simulink model "control_f86_LQR"  (R2019b)
settings: Solver=VariableStepAuto  StartTime=0.0  StopTime=simtime  RelTol=1e-3
values from neighbouring files (symbols this model uses):
  matrices = matrices_generator(linearization,simtime,T,WIND)    [main.m]    (also in matrices.mat = )
  path =     [path.mat]
  T = 0.021    [main.m]
settings Model: Creator=Usuario  LastModifiedBy=Usuario
settings SolverCC: ZeroCrossAlgorithm=Adaptive  AlgebraicLoopSolver=LineSearch
settings DebuggingCC: MaxConsecutiveZCsMsg=none  IgnoredZcDiagnostic=none  UnderSpecifiedDimensionMsg=warning

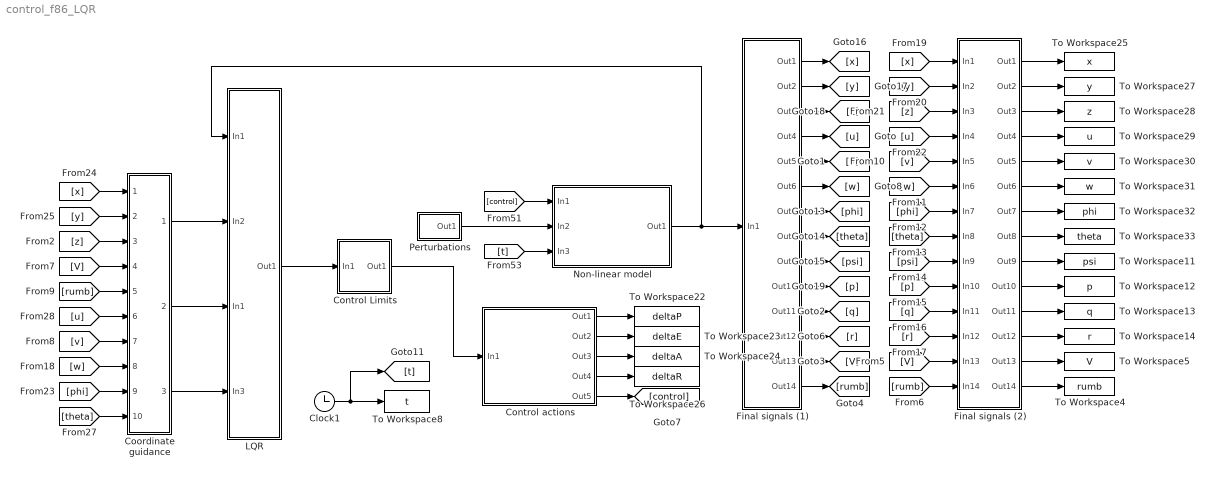
== system control_f86_LQR ==
  Clock1 : Clock
  Control Limits : Subsystem
  Control actions : Subsystem
  Coordinate guidance : Subsystem
  Final signals (1) : Subsystem
  Final signals (2) : Subsystem
  LQR : Subsystem
  Non-linear model : Subsystem
  "Perturbations " : Subsystem
  To Workspace11 : ToWorkspace  VariableName=psi  SampleTime=T
  To Workspace12 : ToWorkspace  VariableName=p  SampleTime=T
  To Workspace13 : ToWorkspace  VariableName=q  SampleTime=T
  To Workspace14 : ToWorkspace  VariableName=r  SampleTime=T
  To Workspace22 : ToWorkspace  VariableName=deltaP  SampleTime=T
  To Workspace23 : ToWorkspace  VariableName=deltaE  SampleTime=T
  To Workspace24 : ToWorkspace  VariableName=deltaA  SampleTime=T
  To Workspace25 : ToWorkspace  VariableName=x  SampleTime=T
  To Workspace26 : ToWorkspace  VariableName=deltaR  SampleTime=T
  To Workspace27 : ToWorkspace  VariableName=y  SampleTime=T
  To Workspace28 : ToWorkspace  VariableName=z  SampleTime=T
  To Workspace29 : ToWorkspace  VariableName=u  SampleTime=T
  To Workspace30 : ToWorkspace  VariableName=v  SampleTime=T
  To Workspace31 : ToWorkspace  VariableName=w  SampleTime=T
  To Workspace32 : ToWorkspace  VariableName=phi  SampleTime=T
  To Workspace33 : ToWorkspace  VariableName=theta  SampleTime=T
  To Workspace4 : ToWorkspace  VariableName=rumb  SampleTime=T
  To Workspace5 : ToWorkspace  VariableName=V  SampleTime=T
  To Workspace8 : ToWorkspace  VariableName=t  SampleTime=T
  wires:
  Non-linear model/1(Out1) -> LQR/1("In1 "), Final signals (1)/1(In1)
  "Perturbations "/1(Out1) -> Non-linear model/2(In2)
  Clock1/1 -> [t], To Workspace8/1
  [control] -> Non-linear model/1(In1)
  [t] -> Non-linear model/3(In3)
  LQR/1(Out1) -> Control Limits/1(In1)
  Control Limits/1(Out1) -> Control actions/1(In1)
  [x] -> Coordinate guidance/1(In1)
  [y] -> Coordinate guidance/2(In2)
  Coordinate guidance/1(Out1) -> LQR/2(In2)
  Coordinate guidance/2(Out2) -> LQR/3(In1)
  Coordinate guidance/3(Out3) -> LQR/4(In3)
  Final signals (2)/10(Out10) -> To Workspace12/1
  Final signals (1)/7(Out7) -> [phi]
  [phi] -> Final signals (2)/7(In7)
  [theta] -> Final signals (2)/8(In8)
  Final signals (2)/1(Out1) -> To Workspace25/1
  [u] -> Final signals (2)/4(In4)
  [r] -> Final signals (2)/12(In12)
  [z] -> Final signals (2)/3(In3)
  Final signals (2)/6(Out6) -> To Workspace31/1
  Final signals (2)/7(Out7) -> To Workspace32/1
  [psi] -> Final signals (2)/9(In9)
  Final signals (2)/9(Out9) -> To Workspace11/1
  Final signals (2)/12(Out12) -> To Workspace14/1
  [V] -> Final signals (2)/13(In13)
  Final signals (1)/1(Out1) -> [x]
  [w] -> Final signals (2)/6(In6)
  [p] -> Final signals (2)/10(In10)
  Final signals (1)/13(Out13) -> [V]
  Final signals (2)/11(Out11) -> To Workspace13/1
  Final signals (2)/8(Out8) -> To Workspace33/1
  Final signals (1)/5(Out5) -> [v]
  Final signals (1)/11(Out11) -> [q]
  Final signals (2)/3(Out3) -> To Workspace28/1
  Final signals (2)/14(Out14) -> To Workspace4/1
  Final signals (1)/9(Out9) -> [psi]
  Final signals (2)/4(Out4) -> To Workspace29/1
  [x] -> Final signals (2)/1(In1)
  [y] -> Final signals (2)/2(In2)
  Final signals (1)/3(Out3) -> [z]
  Final signals (1)/4(Out4) -> [u]
  [rumb] -> Final signals (2)/14(In14)
  [v] -> Final signals (2)/5(In5)
  Final signals (1)/6(Out6) -> [w]
  Final signals (2)/5(Out5) -> To Workspace30/1
  Final signals (1)/14(Out14) -> [rumb]
  Final signals (1)/12(Out12) -> [r]
  Final signals (1)/10(Out10) -> [p]
  Final signals (2)/13(Out13) -> To Workspace5/1
  Final signals (2)/2(Out2) -> To Workspace27/1
  Final signals (1)/8(Out8) -> [theta]
  Final signals (1)/2(Out2) -> [y]
  [q] -> Final signals (2)/11(In11)
  Control actions/5(Out5) -> [control]
  Control actions/1(Out1) -> To Workspace22/1
  Control actions/2(Out2) -> To Workspace23/1
  Control actions/4(Out4) -> To Workspace26/1
  Control actions/3(Out3) -> To Workspace24/1
  [V] -> Coordinate guidance/4(In4)
  [rumb] -> Coordinate guidance/5(In5)
  [u] -> Coordinate guidance/6(In6)
  [v] -> Coordinate guidance/7(In7)
  [w] -> Coordinate guidance/8(In8)
  [phi] -> Coordinate guidance/9(In9)
  [theta] -> Coordinate guidance/10(In10)
  [z] -> Coordinate guidance/3(In3)

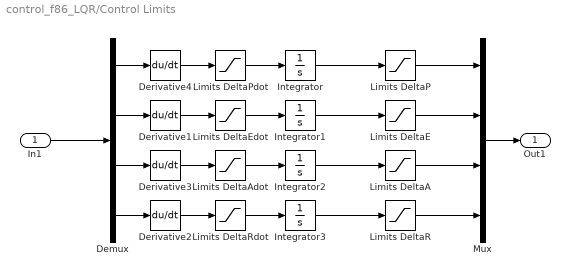
== system control_f86_LQR/Control Limits ==
  In1 : Inport
  Demux : Demux
  Derivative1 : Derivative  CoefficientInTFapproximation=100
  Derivative2 : Derivative  CoefficientInTFapproximation=100
  Derivative3 : Derivative  CoefficientInTFapproximation=100
  Derivative4 : Derivative  CoefficientInTFapproximation=1
  Integrator{,1..3} (4 alike) : Integrator
  Limits DeltaA : Saturate  UpperLimit=matrices.maxdeltaA-matrices.v_0trim(25)  LowerLimit=matrices.mindeltaA-matrices.v_0trim(25)  ZeroCross=off
  Limits DeltaAdot : Saturate  UpperLimit=matrices.maxdeltaAdot  LowerLimit=-matrices.maxdeltaAdot  ZeroCross=off
  Limits DeltaE : Saturate  UpperLimit=matrices.maxdeltaE-matrices.v_0trim(24)  LowerLimit=matrices.mindeltaE-matrices.v_0trim(24)  ZeroCross=off
  Limits DeltaEdot : Saturate  UpperLimit=matrices.maxdeltaEdot  LowerLimit=-matrices.maxdeltaEdot  ZeroCross=off
  Limits DeltaP : Saturate  UpperLimit=matrices.maxdeltaP-matrices.v_0trim(23)  LowerLimit=matrices.mindeltaP-matrices.v_0trim(23)  ZeroCross=off
  Limits DeltaPdot : Saturate  UpperLimit=matrices.maxdeltaPdot  LowerLimit=-matrices.maxdeltaPdot  ZeroCross=off
  Limits DeltaR : Saturate  UpperLimit=matrices.maxdeltaR-matrices.v_0trim(26)  LowerLimit=matrices.mindeltaR-matrices.v_0trim(26)  ZeroCross=off
  Limits DeltaRdot : Saturate  UpperLimit=matrices.maxdeltaRdot  LowerLimit=-matrices.maxdeltaRdot  ZeroCross=off
  Mux : Mux
  Out1 : Outport
  wires:
  In1/1 -> Demux/1
  Mux/1 -> Out1/1
  Demux/4 -> Derivative2/1
  Limits DeltaEdot/1 -> Integrator1/1
  Demux/3 -> Derivative3/1
  Integrator3/1 -> Limits DeltaR/1
  Limits DeltaP/1 -> Mux/1
  Demux/2 -> Derivative1/1
  Limits DeltaR/1 -> Mux/4
  Integrator/1 -> Limits DeltaP/1
  Limits DeltaAdot/1 -> Integrator2/1
  Derivative3/1 -> Limits DeltaAdot/1
  Limits DeltaRdot/1 -> Integrator3/1
  Limits DeltaPdot/1 -> Integrator/1
  Derivative2/1 -> Limits DeltaRdot/1
  Integrator2/1 -> Limits DeltaA/1
  Demux/1 -> Derivative4/1
  Derivative4/1 -> Limits DeltaPdot/1
  Derivative1/1 -> Limits DeltaEdot/1
  Limits DeltaA/1 -> Mux/3
  Limits DeltaE/1 -> Mux/2
  Integrator1/1 -> Limits DeltaE/1

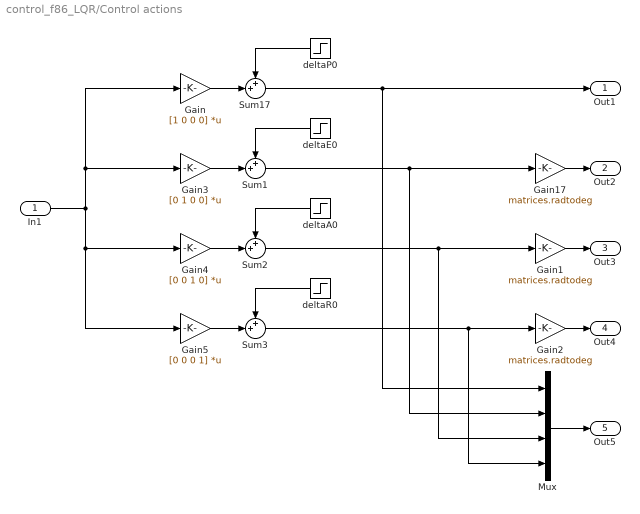
== system control_f86_LQR/Control actions ==
  In1 : Inport
  Gain : Gain  Gain=[1 0 0 0]  Multiplication=Matrix(K*u)
  Gain1 : Gain  Gain=matrices.radtodeg
  Gain17 : Gain  Gain=matrices.radtodeg
  Gain2 : Gain  Gain=matrices.radtodeg
  Gain3 : Gain  Gain=[0 1 0 0]  Multiplication=Matrix(K*u)
  Gain4 : Gain  Gain=[0 0 1 0]  Multiplication=Matrix(K*u)
  Gain5 : Gain  Gain=[0 0 0 1]  Multiplication=Matrix(K*u)
  Mux : Mux
  Sum{1..3,17} (4 alike) : Sum  Inputs=++|
  deltaA0 : Step  Time=0  After=matrices.v_0trim(25)  SampleTime=T
  deltaE0 : Step  Time=0  After=matrices.v_0trim(24)  SampleTime=T
  deltaP0 : Step  Time=0  After=matrices.v_0trim(23)  SampleTime=T
  deltaR0 : Step  Time=0  After=matrices.v_0trim(26)  SampleTime=T
  Out1 : Outport
  Out2 : Outport  Port=2
  Out3 : Outport  Port=3
  Out4 : Outport  Port=4
  Out5 : Outport  Port=5
  wires:
  In1/1 -> Gain5/1, Gain4/1, Gain3/1, Gain/1
  Sum17/1 -> Mux/1, Out1/1
  deltaP0/1 -> Sum17/1
  deltaE0/1 -> Sum1/1
  deltaA0/1 -> Sum2/1
  deltaR0/1 -> Sum3/1
  Sum1/1 -> Mux/2, Gain17/1
  Gain17/1 -> Out2/1
  Gain1/1 -> Out3/1
  Sum2/1 -> Mux/3, Gain1/1
  Gain2/1 -> Out4/1
  Sum3/1 -> Mux/4, Gain2/1
  Gain/1 -> Sum17/2
  Gain3/1 -> Sum1/2
  Gain4/1 -> Sum2/2
  Gain5/1 -> Sum3/2
  Mux/1 -> Out5/1

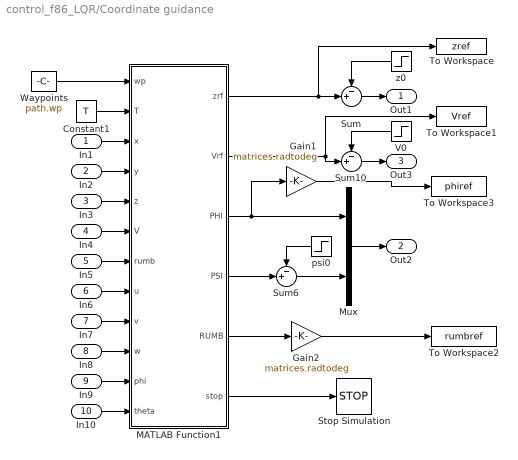
== system control_f86_LQR/Coordinate guidance ==
  In1 : Inport
  In2 : Inport  Port=2
  In3 : Inport  Port=3
  In4 : Inport  Port=4
  In5 : Inport  Port=5
  In6 : Inport  Port=6
  In7 : Inport  Port=7
  In8 : Inport  Port=8
  In9 : Inport  Port=9
  In10 : Inport  Port=10
  Constant1 : Constant  Value=T  SampleTime=T
  Gain1 : Gain  Gain=matrices.radtodeg
  Gain2 : Gain  Gain=matrices.radtodeg
  MATLAB Function1 : MATLAB Function  TreatAsAtomicUnit=on  SystemSampleTime=T
  Mux : Mux  Inputs=2
  Stop Simulation : Stop
  Sum : Sum  Inputs=-+|
  Sum10 : Sum  Inputs=-+|
  Sum6 : Sum  Inputs=-+|
  To Workspace : ToWorkspace  VariableName=zref  SampleTime=T
  To Workspace1 : ToWorkspace  VariableName=Vref  SampleTime=T
  To Workspace2 : ToWorkspace  VariableName=rumbref  SampleTime=T
  To Workspace3 : ToWorkspace  VariableName=phiref  SampleTime=T
  V0 : Step  Time=0  After=matrices.v_0trim(11)  SampleTime=T
  Waypoints : Constant  Value=path.wp  OutDataTypeStr=double  SampleTime=T
  psi0 : Step  Time=0  After=matrices.v_0trim(7)  SampleTime=T
  z0 : Step  Time=0  After=matrices.v_0trim(1)  SampleTime=T
  Out1 : Outport
  Out2 : Outport  Port=2
  Out3 : Outport  Port=3
  wires:
  Gain1/1 -> To Workspace3/1
  MATLAB Function1/3(PHI) -> Gain1/1, Mux/1
  MATLAB Function1/5(RUMB) -> Gain2/1
  Constant1/1 -> MATLAB Function1/2(T)
  In1/1 -> MATLAB Function1/3(x)
  In2/1 -> MATLAB Function1/4(y)
  Waypoints/1 -> MATLAB Function1/1(wp)
  MATLAB Function1/1(zrf) -> Sum/2, To Workspace/1
  Mux/1 -> Out2/1
  z0/1 -> Sum/1
  Sum/1 -> Out1/1
  V0/1 -> Sum10/1
  Sum10/1 -> Out3/1
  MATLAB Function1/2(Vrf) -> To Workspace1/1, Sum10/2
  psi0/1 -> Sum6/1
  Sum6/1 -> Mux/2
  MATLAB Function1/4(PSI) -> Sum6/2
  In10/1 -> MATLAB Function1/12(theta)
  In9/1 -> MATLAB Function1/11(phi)
  In8/1 -> MATLAB Function1/10(w)
  In7/1 -> MATLAB Function1/9(v)
  In6/1 -> MATLAB Function1/8(u)
  In5/1 -> MATLAB Function1/7(rumb)
  In4/1 -> MATLAB Function1/6(V)
  In3/1 -> MATLAB Function1/5(z)
  MATLAB Function1/6(stop) -> Stop Simulation/1
  Gain2/1 -> To Workspace2/1

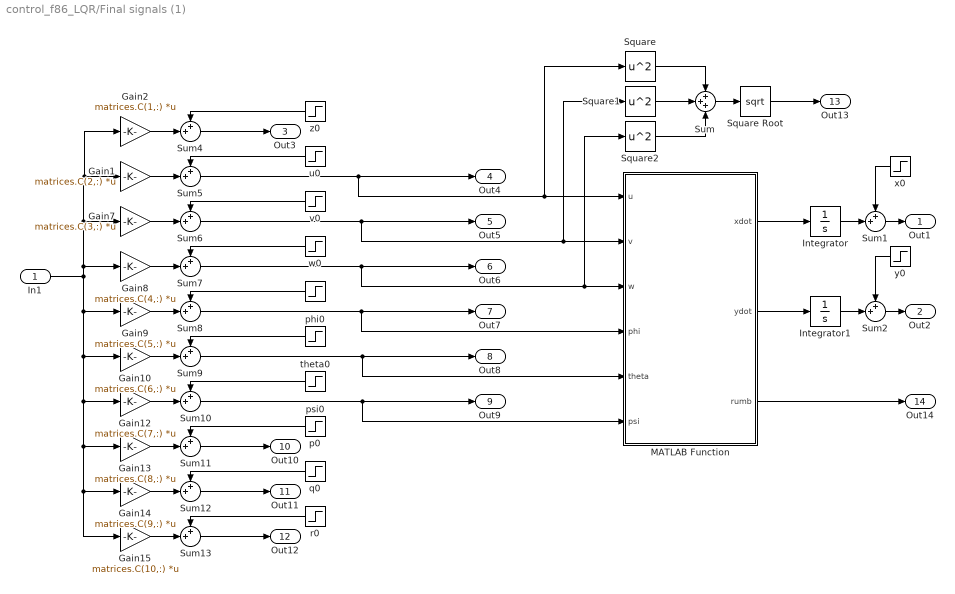
== system control_f86_LQR/Final signals (1) ==
  In1 : Inport
  Gain1 : Gain  Gain=matrices.C(2,:)  Multiplication=Matrix(K*u)
  Gain10 : Gain  Gain=matrices.C(6,:)  Multiplication=Matrix(K*u)
  Gain12 : Gain  Gain=matrices.C(7,:)  Multiplication=Matrix(K*u)
  Gain13 : Gain  Gain=matrices.C(8,:)  Multiplication=Matrix(K*u)
  Gain14 : Gain  Gain=matrices.C(9,:)  Multiplication=Matrix(K*u)
  Gain15 : Gain  Gain=matrices.C(10,:)  Multiplication=Matrix(K*u)
  Gain2 : Gain  Gain=matrices.C(1,:)  Multiplication=Matrix(K*u)
  Gain7 : Gain  Gain=matrices.C(3,:)  Multiplication=Matrix(K*u)
  Gain8 : Gain  Gain=matrices.C(4,:)  Multiplication=Matrix(K*u)
  Gain9 : Gain  Gain=matrices.C(5,:)  Multiplication=Matrix(K*u)
  Integrator : Integrator
  Integrator1 : Integrator
  MATLAB Function : MATLAB Function  TreatAsAtomicUnit=on
  Square : Math  Operator=square  SignedPower=off  SaturateOnIntegerOverflow=on
  Square Root : Sqrt  SaturateOnIntegerOverflow=on
  Square1 : Math  Operator=square  SignedPower=off  SaturateOnIntegerOverflow=on
  Square2 : Math  Operator=square  SignedPower=off  SaturateOnIntegerOverflow=on
  Sum : Sum  Inputs=+++
  Sum{1..2,4..13} (12 alike) : Sum  Inputs=++|
  p0 : Step  Time=0  After=matrices.v_0trim(8)  SampleTime=T
  phi0 : Step  Time=0  After=matrices.v_0trim(5)  SampleTime=T
  psi0 : Step  Time=0  After=matrices.v_0trim(7)  SampleTime=T
  q0 : Step  Time=0  After=matrices.v_0trim(9)  SampleTime=T
  r0 : Step  Time=0  After=matrices.v_0trim(10)  SampleTime=T
  theta0 : Step  Time=0  After=matrices.v_0trim(6)  SampleTime=T
  u0 : Step  Time=0  After=matrices.v_0trim(2)  SampleTime=T
  v0 : Step  Time=0  After=matrices.v_0trim(3)  SampleTime=T
  w0 : Step  Time=0  After=matrices.v_0trim(4)  SampleTime=T
  x0 : Step  Time=0  After=path.wp(1,1)  SampleTime=T
  y0 : Step  Time=0  After=path.wp(1,2)  SampleTime=T
  z0 : Step  Time=0  After=matrices.v_0trim(1)  SampleTime=T
  Out1 : Outport
  Out2 : Outport  Port=2
  Out3 : Outport  Port=3
  Out4 : Outport  Port=4
  Out5 : Outport  Port=5
  Out6 : Outport  Port=6
  Out7 : Outport  Port=7
  Out8 : Outport  Port=8
  Out9 : Outport  Port=9
  Out10 : Outport  Port=10
  Out11 : Outport  Port=11
  Out12 : Outport  Port=12
  Out13 : Outport  Port=13
  Out14 : Outport  Port=14
  wires:
  Sum13/1 -> Out12/1
  Sum4/1 -> Out3/1
  Sum11/1 -> Out10/1
  Sum12/1 -> Out11/1
  Sum9/1 -> MATLAB Function/5(theta), Out8/1
  Sum8/1 -> MATLAB Function/4(phi), Out7/1
  Sum10/1 -> MATLAB Function/6(psi), Out9/1
  z0/1 -> Sum4/1
  u0/1 -> Sum5/1
  v0/1 -> Sum6/1
  w0/1 -> Sum7/1
  phi0/1 -> Sum8/1
  theta0/1 -> Sum9/1
  psi0/1 -> Sum10/1
  p0/1 -> Sum11/1
  q0/1 -> Sum12/1
  r0/1 -> Sum13/1
  In1/1 -> Gain12/1, Gain13/1, Gain14/1, Gain15/1, Gain10/1, Gain9/1, Gain8/1, Gain7/1, Gain2/1, Gain1/1
  MATLAB Function/3(rumb) -> Out14/1
  Square1/1 -> Sum/2
  Square2/1 -> Sum/3
  Sum/1 -> Square Root/1
  Square/1 -> Sum/1
  Square Root/1 -> Out13/1
  Sum6/1 -> Out5/1, Square1/1, MATLAB Function/2(v)
  Sum5/1 -> Out4/1, Square/1, MATLAB Function/1(u)
  Sum7/1 -> Out6/1, Square2/1, MATLAB Function/3(w)
  MATLAB Function/1(xdot) -> Integrator/1
  MATLAB Function/2(ydot) -> Integrator1/1
  Gain15/1 -> Sum13/2
  Gain14/1 -> Sum12/2
  Gain13/1 -> Sum11/2
  Gain12/1 -> Sum10/2
  Gain10/1 -> Sum9/2
  Gain9/1 -> Sum8/2
  Gain8/1 -> Sum7/2
  Gain7/1 -> Sum6/2
  Gain1/1 -> Sum5/2
  Gain2/1 -> Sum4/2
  Sum1/1 -> Out1/1
  Sum2/1 -> Out2/1
  x0/1 -> Sum1/1
  y0/1 -> Sum2/1
  Integrator/1 -> Sum1/2
  Integrator1/1 -> Sum2/2

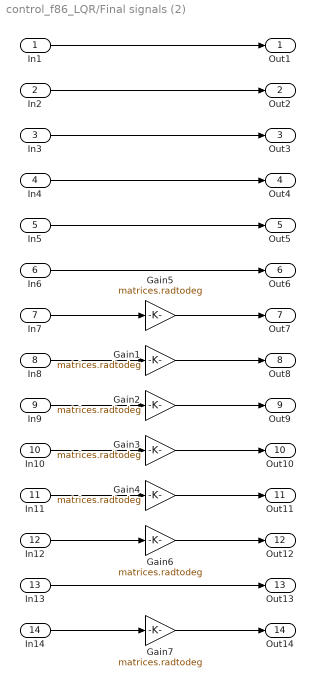
== system control_f86_LQR/Final signals (2) ==
  In1 : Inport
  In2 : Inport  Port=2
  In3 : Inport  Port=3
  In4 : Inport  Port=4
  In5 : Inport  Port=5
  In6 : Inport  Port=6
  In7 : Inport  Port=7
  In8 : Inport  Port=8
  In9 : Inport  Port=9
  In10 : Inport  Port=10
  In11 : Inport  Port=11
  In12 : Inport  Port=12
  In13 : Inport  Port=13
  In14 : Inport  Port=14
  Gain{1..7} (7 alike) : Gain  Gain=matrices.radtodeg
  Out1 : Outport
  Out2 : Outport  Port=2
  Out3 : Outport  Port=3
  Out4 : Outport  Port=4
  Out5 : Outport  Port=5
  Out6 : Outport  Port=6
  Out7 : Outport  Port=7
  Out8 : Outport  Port=8
  Out9 : Outport  Port=9
  Out10 : Outport  Port=10
  Out11 : Outport  Port=11
  Out12 : Outport  Port=12
  Out13 : Outport  Port=13
  Out14 : Outport  Port=14
  wires:
  In1/1 -> Out1/1
  In2/1 -> Out2/1
  In3/1 -> Out3/1
  In4/1 -> Out4/1
  In5/1 -> Out5/1
  In6/1 -> Out6/1
  Gain5/1 -> Out7/1
  Gain1/1 -> Out8/1
  Gain2/1 -> Out9/1
  Gain3/1 -> Out10/1
  Gain4/1 -> Out11/1
  Gain6/1 -> Out12/1
  In12/1 -> Gain6/1
  In11/1 -> Gain4/1
  In10/1 -> Gain3/1
  In9/1 -> Gain2/1
  In8/1 -> Gain1/1
  In7/1 -> Gain5/1
  In14/1 -> Gain7/1
  Gain7/1 -> Out14/1
  In13/1 -> Out13/1

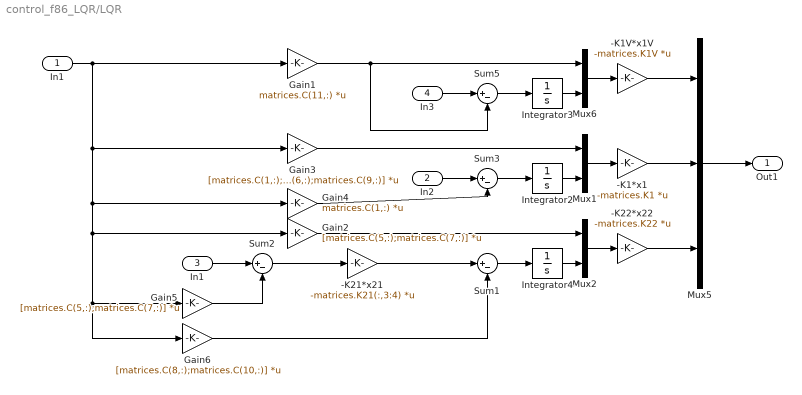
== system control_f86_LQR/LQR ==
  "In1 " : Inport
  In2 : Inport  Port=2
  In1 : Inport  Port=3
  In3 : Inport  Port=4
  -K1*x1 : Gain  Gain=-matrices.K1  Multiplication=Matrix(K*u)
  -K1V*x1V : Gain  Gain=-matrices.K1V  Multiplication=Matrix(K*u)
  -K21*x21 : Gain  Gain=-matrices.K21(:,3:4)  Multiplication=Matrix(K*u)
  -K22*x22 : Gain  Gain=-matrices.K22  Multiplication=Matrix(K*u)
  Gain1 : Gain  Gain=matrices.C(11,:)  Multiplication=Matrix(K*u)
  Gain2 : Gain  Gain=[matrices.C(5,:);matrices.C(7,:)]  Multiplication=Matrix(K*u)
  Gain3 : Gain  Gain=[matrices.C(1,:);matrices.C(2,:);matrices.C(4,:);matrices.C(6,:);matrices.C(9,:)]  Multiplication=Matrix(K*u)
  Gain4 : Gain  Gain=matrices.C(1,:)  Multiplication=Matrix(K*u)
  Gain5 : Gain  Gain=[matrices.C(5,:);matrices.C(7,:)]  Multiplication=Matrix(K*u)
  Gain6 : Gain  Gain=[matrices.C(8,:);matrices.C(10,:)]  Multiplication=Matrix(K*u)
  Integrator2 : Integrator
  Integrator3 : Integrator
  Integrator4 : Integrator
  Mux1 : Mux  Inputs=2
  Mux2 : Mux  Inputs=2
  Mux5 : Mux  Inputs=3
  Mux6 : Mux  Inputs=2
  Sum{1..3,5} (4 alike) : Sum  Inputs=|+-
  Out1 : Outport
  wires:
  Mux6/1 -> -K1V*x1V/1
  Sum5/1 -> Integrator3/1
  Integrator3/1 -> Mux6/2
  Integrator2/1 -> Mux1/2
  Sum3/1 -> Integrator2/1
  Mux1/1 -> -K1*x1/1
  Mux5/1 -> Out1/1
  -K1*x1/1 -> Mux5/2
  -K1V*x1V/1 -> Mux5/1
  Gain3/1 -> Mux1/1
  Sum1/1 -> Integrator4/1
  Integrator4/1 -> Mux2/2
  -K22*x22/1 -> Mux5/3
  Mux2/1 -> -K22*x22/1
  Gain2/1 -> Mux2/1
  In2/1 -> Sum3/1
  Gain1/1 -> Mux6/1, Sum5/2
  Gain4/1 -> Sum3/2
  Gain5/1 -> Sum2/2
  In1/1 -> Sum2/1
  In3/1 -> Sum5/1
  Gain6/1 -> Sum1/2
  "In1 "/1 -> Gain4/1, Gain6/1, Gain5/1, Gain2/1, Gain3/1, Gain1/1
  -K21*x21/1 -> Sum1/1
  Sum2/1 -> -K21*x21/1

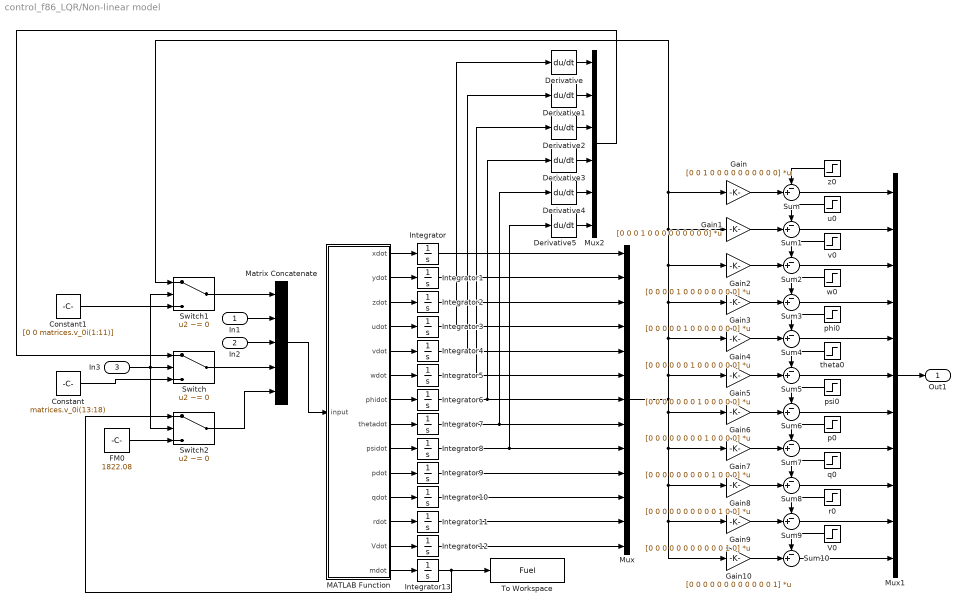
== system control_f86_LQR/Non-linear model ==
  In1 : Inport
  In2 : Inport  Port=2
  In3 : Inport  Port=3
  Constant : Constant  Value=matrices.v_0i(13:18)  SampleTime=T
  Constant1 : Constant  Value=[0 0 matrices.v_0i(1:11)]  SampleTime=T
  Derivative{,1..5} (6 alike) : Derivative
  FM0 : Constant  Value=1822.08  SampleTime=T
  Gain : Gain  Gain=[0 0 1 0 0 0 0 0 0 0 0 0 0]  Multiplication=Matrix(K*u)
  Gain1 : Gain  Gain=[0 0 0 1 0 0 0 0 0 0 0 0 0]  Multiplication=Matrix(K*u)
  Gain10 : Gain  Gain=[0 0 0 0 0 0 0 0 0 0 0 0 1]  Multiplication=Matrix(K*u)
  Gain2 : Gain  Gain=[0 0 0 0 1 0 0 0 0 0 0 0 0]  Multiplication=Matrix(K*u)
  Gain3 : Gain  Gain=[0 0 0 0 0 1 0 0 0 0 0 0 0]  Multiplication=Matrix(K*u)
  Gain4 : Gain  Gain=[0 0 0 0 0 0 1 0 0 0 0 0 0]  Multiplication=Matrix(K*u)
  Gain5 : Gain  Gain=[0 0 0 0 0 0 0 1 0 0 0 0 0]  Multiplication=Matrix(K*u)
  Gain6 : Gain  Gain=[0 0 0 0 0 0 0 0 1 0 0 0 0]  Multiplication=Matrix(K*u)
  Gain7 : Gain  Gain=[0 0 0 0 0 0 0 0 0 1 0 0 0]  Multiplication=Matrix(K*u)
  Gain8 : Gain  Gain=[0 0 0 0 0 0 0 0 0 0 1 0 0]  Multiplication=Matrix(K*u)
  Gain9 : Gain  Gain=[0 0 0 0 0 0 0 0 0 0 0 1 0]  Multiplication=Matrix(K*u)
  Integrator : Integrator
  Integrator1 : Integrator
  Integrator10 : Integrator  InitialCondition=matrices.v_0i(9)
  Integrator11 : Integrator  InitialCondition=matrices.v_0i(10)
  Integrator12 : Integrator  InitialCondition=matrices.v_0i(11)
  Integrator13 : Integrator  InitialCondition=1822.08
  Integrator2 : Integrator  InitialCondition=matrices.v_0i(1)
  Integrator3 : Integrator  InitialCondition=matrices.v_0i(2)
  Integrator4 : Integrator  InitialCondition=matrices.v_0i(3)
  Integrator5 : Integrator  InitialCondition=matrices.v_0i(4)
  Integrator6 : Integrator  InitialCondition=matrices.v_0i(5)
  Integrator7 : Integrator  InitialCondition=matrices.v_0i(6)
  Integrator8 : Integrator  InitialCondition=matrices.v_0i(7)
  Integrator9 : Integrator  InitialCondition=matrices.v_0i(8)
  MATLAB Function : MATLAB Function  TreatAsAtomicUnit=on
  Matrix Concatenate : Concatenate  NumInputs=5
  Mux : Mux  Inputs=13
  Mux1 : Mux  Inputs=11
  Mux2 : Mux  Inputs=6
  Sum{,1..10} (11 alike) : Sum  Inputs=-+|
  Switch : Switch  Criteria=u2 ~= 0
  Switch1 : Switch  Criteria=u2 ~= 0
  Switch2 : Switch  Criteria=u2 ~= 0
  To Workspace : ToWorkspace  VariableName=Fuel  SampleTime=T
  V0 : Step  Time=0  After=matrices.v_0trim(11)  SampleTime=T
  p0 : Step  Time=0  After=matrices.v_0trim(8)  SampleTime=T
  phi0 : Step  Time=0  After=matrices.v_0trim(5)  SampleTime=T
  psi0 : Step  Time=0  After=matrices.v_0trim(7)  SampleTime=T
  q0 : Step  Time=0  After=matrices.v_0trim(9)  SampleTime=T
  r0 : Step  Time=0  After=matrices.v_0trim(10)  SampleTime=T
  theta0 : Step  Time=0  After=matrices.v_0trim(6)  SampleTime=T
  u0 : Step  Time=0  After=matrices.v_0trim(2)  SampleTime=T
  v0 : Step  Time=0  After=matrices.v_0trim(3)  SampleTime=T
  w0 : Step  Time=0  After=matrices.v_0trim(4)  SampleTime=T
  z0 : Step  Time=0  After=matrices.v_0trim(1)  SampleTime=T
  Out1 : Outport
  wires:
  Integrator10/1 -> Mux/11
  Integrator12/1 -> Mux/13
  Integrator11/1 -> Mux/12
  Integrator7/1 -> Derivative4/1, Mux/8
  Integrator6/1 -> Derivative3/1, Mux/7
  Integrator8/1 -> Derivative5/1, Mux/9
  Integrator9/1 -> Mux/10
  Integrator2/1 -> Mux/3
  Integrator/1 -> Mux/1
  Integrator5/1 -> Mux/6, Derivative2/1
  Integrator3/1 -> Mux/4, Derivative/1
  Integrator1/1 -> Mux/2
  MATLAB Function/9(psidot) -> Integrator8/1
  MATLAB Function/10(pdot) -> Integrator9/1
  MATLAB Function/12(rdot) -> Integrator11/1
  MATLAB Function/5(vdot) -> Integrator4/1
  MATLAB Function/3(zdot) -> Integrator2/1
  Integrator4/1 -> Mux/5, Derivative1/1
  MATLAB Function/2(ydot) -> Integrator1/1
  MATLAB Function/11(qdot) -> Integrator10/1
  MATLAB Function/1(xdot) -> Integrator/1
  MATLAB Function/7(phidot) -> Integrator6/1
  MATLAB Function/8(thetadot) -> Integrator7/1
  MATLAB Function/13(Vdot) -> Integrator12/1
  MATLAB Function/4(udot) -> Integrator3/1
  MATLAB Function/6(wdot) -> Integrator5/1
  In2/1 -> Matrix Concatenate/3
  Switch/1 -> Matrix Concatenate/4
  In3/1 -> Switch/2, Switch2/2, Switch1/2
  Switch1/1 -> Matrix Concatenate/1
  Matrix Concatenate/1 -> MATLAB Function/1(input)
  Constant1/1 -> Switch1/3
  Constant/1 -> Switch/3
  Mux2/1 -> Switch/1
  Derivative/1 -> Mux2/1
  Derivative1/1 -> Mux2/2
  Derivative2/1 -> Mux2/3
  In1/1 -> Matrix Concatenate/2
  z0/1 -> Sum/1
  u0/1 -> Sum1/1
  v0/1 -> Sum2/1
  w0/1 -> Sum3/1
  phi0/1 -> Sum4/1
  theta0/1 -> Sum5/1
  psi0/1 -> Sum6/1
  p0/1 -> Sum7/1
  q0/1 -> Sum8/1
  r0/1 -> Sum9/1
  V0/1 -> Sum10/1
  Sum/1 -> Mux1/1
  Sum1/1 -> Mux1/2
  Sum2/1 -> Mux1/3
  Sum3/1 -> Mux1/4
  Sum4/1 -> Mux1/5
  Sum5/1 -> Mux1/6
  Sum6/1 -> Mux1/7
  Sum7/1 -> Mux1/8
  Sum8/1 -> Mux1/9
  Sum9/1 -> Mux1/10
  Sum10/1 -> Mux1/11
  Mux1/1 -> Out1/1
  Derivative3/1 -> Mux2/4
  Derivative4/1 -> Mux2/5
  Derivative5/1 -> Mux2/6
  Gain/1 -> Sum/2
  Gain1/1 -> Sum1/2
  Gain2/1 -> Sum2/2
  Gain3/1 -> Sum3/2
  Gain4/1 -> Sum4/2
  Gain5/1 -> Sum5/2
  Gain6/1 -> Sum6/2
  Gain7/1 -> Sum7/2
  Mux/1 -> Gain6/1, Gain7/1, Gain8/1, Gain9/1, Gain10/1, Gain5/1, Gain4/1, Gain3/1, Gain2/1, Gain1/1, Gain/1, Switch1/1
  Gain8/1 -> Sum8/2
  Gain9/1 -> Sum9/2
  Gain10/1 -> Sum10/2
  FM0/1 -> Switch2/3
  MATLAB Function/14(mdot) -> Integrator13/1
  Integrator13/1 -> To Workspace/1, Switch2/1
  Switch2/1 -> Matrix Concatenate/5

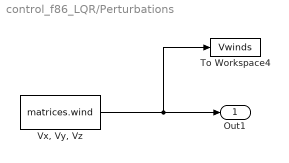
== system control_f86_LQR/Perturbations  ==
  To Workspace4 : ToWorkspace  VariableName=Vwinds  SampleTime=T
  "Vx, Vy, Vz" : FromWorkspace  VariableName=matrices.wind  SampleTime=T
  Out1 : Outport
  wires:
  "Vx, Vy, Vz"/1 -> To Workspace4/1, Out1/1

== matlab function control_f86_LQR/Coordinate guidance/MATLAB Function1 ==
  data: wp input; T input; x input; y input; z input; V input; rumb input; u input; v input; w input; phi input; theta input; zrf output; Vrf output; PHI output; PSI output; RUMB output; stop output
function [zrf,Vrf,PHI,PSI,RUMB,stop] = guidance(wp,T,x,y,z,V,rumb,u,v,w,phi,theta)

L = 0.5*(2*V^2/(9.81*sqrt(5.5^2-1)));

err  = abs((wp(:,1)-x).^2+(wp(:,2)-y).^2-L^2);
err2 = sort(err);

a = 0;
b = 0;
c = 0;
d = 0;

for i = 1:length(err)
    if (err(i) == err2(1))
        a = i;
    elseif (err(i) == err2(2))
        b = i;
    elseif (err(i) == err2(3))
        c = i;
    elseif (err(i) == err2(4))
        d = i;
    end
end

MAX = max(max(a,b),max(c,d));

if MAX > size(wp,1)
    MAX = size(wp,1);
end

xrf   = wp(MAX,1);
yrf   = wp(MAX,2);

err_2  = abs((wp(:,1)-x).^2+(wp(:,2)-y).^2-50);
err2_2 = sort(err_2);

a_2 = 0;
b_2 = 0;
c_2 = 0;
d_2 = 0;

for i = 1:length(err2_2)
    if (err_2(i) == err2_2(1))
        a_2 = i;
    elseif (err_2(i) == err2_2(2))
        b_2 = i;
    elseif (err_2(i) == err2_2(3))
        c_2 = i;
    elseif (err_2(i) == err2_2(4))
        d_2 = i;
    end
end
MAX2  = max(max(a_2,b_2),max(c_2,d_2));
zrf   = wp(min(MAX2,size(wp,1)),3);
Vrf   = wp(min(MAX2,size(wp,1)),4);
psirf = wp(MAX2,6);
% Zrf=zrf;
% if (abs(psirf) > 3)&&(abs(wp(min(MAX2,size(wp,1)),3)-wp(min(MAX2+1,size(wp,1)),3)) < 0.01)
%     zrf = z+(zrf-z)/(abs(psirf)-1.75);
% end

% if (wp(max(MAX2-100,1),6) ~= 0)||(wp(MAX2,6) ~= 0)||(wp(min(MAX2+100,size(wp,1)),6) ~= 0)
%     dE = 1;
% else
%     dE = 0;
% end

if sqrt((x-wp(end,1))^2+(y-wp(end,2))^2+(z-wp(end,3))^2) < 50
    stop = 1;
else
    stop = 0;
end

% Proportional guiding

Vvector  = [V*cos(rumb) V*sin(rumb)];
distance = [xrf-x yrf-y];
chi      = -atan2(distance(1)*Vvector(2)-distance(2)*Vvector(1),...
           distance(1)*Vvector(1)+distance(2)*Vvector(2));
rumbvar = sign(chi)*2*V/L*T;
% if (abs(psirf) < 0.01)&&(abs(chi)*180/pi < 10)
%     rumbvar = 0;
% end
RUMB    = rumb+rumbvar;

n   = min(sqrt((2*V^2*sin(chi)/(9.81*L))^2+1),5.5);
% if (w < 0)&&(abs(psirf) < 0.01)
%    n = min(sqrt(max((1+w/20),0)*(2*V^2*sin(chi)/(9.81*L))^2+1),5.5);
% end
PHI = sign(chi)*min(acos(1/n),acos(1/5.5));

girophi         = [1,0,0;0,cos(phi),sin(phi);0,(-1).*sin(phi),cos(phi)];
girotheta       = [cos(theta),0,(-1).*sin(theta);0,1,0;sin(theta),0,cos(theta)];
Matrix_rotation = girophi*girotheta; 

V_vect    = [u;v;w]; 

uvw       = transpose(Matrix_rotation)*V_vect;

PSI       = RUMB-atan(uvw(2,1)/uvw(1,1));
% if (w < 0)&&(abs(psirf) < 0.01)
%    PSI    = RUMB-max((1+w/10),0)*atan(uvw(2,1)/uvw(1,1));
% end

end

== matlab function control_f86_LQR/Final signals (1)/MATLAB Function ==
  data: xdot output; ydot output; u input; rumb output; v input; w input; phi input; theta input; psi input
function [xdot,ydot,rumb] =  Dreal(u,v,w,phi,theta,psi)

girophi         = [1,0,0;0,cos(phi),sin(phi);0,(-1).*sin(phi),cos(phi)];
girotheta       = [cos(theta),0,(-1).*sin(theta);0,1,0;sin(theta),0,cos(theta)];
giropsi         = [cos(psi),sin(psi),0;(-1).*sin(psi),cos(psi),0;0,0,1];
Matrix_rotation = girophi*girotheta; 
MBH             = Matrix_rotation*giropsi; % Local horizon axes to body axes

V_vect    = [u;v;w]; 

uvw       = transpose(Matrix_rotation)*V_vect;

rumb      = psi+atan(uvw(2,1)/uvw(1,1));

dxyz      = transpose(MBH)*V_vect;
xdot      = dxyz(1,1);
ydot      = dxyz(2,1);

end

== matlab function control_f86_LQR/Non-linear model/MATLAB Function ==
  data: input input; xdot output; ydot output; zdot output; udot output; vdot output; wdot output; phidot output; thetadot output; psidot output; pdot output; qdot output; rdot output; Vdot output; mdot output
function [xdot,ydot,zdot,udot,vdot,wdot,phidot,thetadot,psidot,pdot,qdot,rdot,Vdot,mdot] = nonlinearmodel(input)

%% Instantaneous values from all variables

z      = input(3,1);
u      = input(4,1);
v      = input(5,1);
w      = input(6,1);
phi    = input(7,1);
theta  = input(8,1);
psi    = input(9,1);
p      = input(10,1);
q      = input(11,1);
r      = input(12,1);
V      = input(13,1);
deltaP = input(14,1);
deltaE = input(15,1);
deltaA = input(16,1);
deltaR = input(17,1);
Vxwind = input(18,1);
Vywind = input(19,1);
Vzwind = input(20,1);
udotref = input(21,1);
vdotref = input(22,1);
wdotref = input(23,1);
phidotref   = input(24,1);
thetadotref = input(25,1);
psidotref   = input(26,1);
FM = input(27,1);

%% Atmospheric conditions

rho_0 = 1.225;
mu_0  = 1.78941*10^(-5);
T_0   = 288.15;
p_0   = 101325;
gamma = 1.4;
R     = 286.9;

P     = p_0*(1+(-0.2257E-4).*z).^0.5256E1;
rho   = rho_0*(1+(-0.2257E-4).*z).^0.4256E1;
T     = T_0*(1+(-0.2257E-4).*z);
mu    = 0.1458E-5.*T.^(3/2).*(0.1104E3+T).^(-1);
a     = sqrt(gamma*R*T);

sigma = rho/rho_0;
thetaT= T/T_0;

%% THRUST MODEL

TSL    = 26289;
Thrust = TSL*(sigma^1.2)*deltaP;
TSFC0  = 2.56*10^(-5);
TSFC   = TSFC0*(sigma^0.1);

%% GEOMETRICAL PARAMETERS

fttomt = 0.3048; %Ft to mts

cwr     = 10.3*fttomt; %Wing
cwt     = 5.3*fttomt;
bw      = 37.1*fttomt;
Sw      = 26.882;
lambdaw = cwt/cwr;
cw      = (2/3)*cwr*(1+lambdaw+lambdaw^2)/(1+lambdaw);
ARw     = bw^2/Sw;
etaMACw = (1/3)*(1+2*lambdaw)/(1+lambdaw);
Yw      = bw/2*etaMACw;
LbdaLEw = 37.5094;

ctr     = 3.8*fttomt; %Horizontal stabilizer
ctt     = 1.7*fttomt;
bt      = 12.8*fttomt;
St      = 3.27;
lambdat = ctt/ctr;
ct      = (2/3)*ctr*(1+lambdat+lambdat^2)/(1+lambdat);
ARt     = bt^2/St;
etaMACt = (1/3)*(1+2*lambdat)/(1+lambdat);
Yt      = bt/2*etaMACt;
LbdaLEt = 38.0337;

Lfuselage = 37.5*fttomt;

hiatus   = 4.00543;

xACw     = Yw*tand(LbdaLEw)+0.25*cw;
xACt     = Yt*tand(LbdaLEt)+0.25*ct+hiatus+cwr;

%% MASS AND INERTIA MOMENT

mdot = -TSFC*Thrust;
m    = 5756.13+FM;
Ixx  = (m-839.18)*(bw/2)^2*0.322^2+3703.73;
Iyy  = (m-839.18)*(Lfuselage/2)^2*0.346^2+87.18;
Izz  = (m-839.18)*((bw+Lfuselage)/2)^2*0.464^2+87.18;
Ixy  = 0;
Iyx  = 0;
Ixz  = 0;
Izx  = 0;
Iyz  = 0;
Izy  = 0;

m0i   = 7578.21;
FM0   = 1822.08;
xcog0 = 2.50; % Gravity center wrt wing apex
xcogf = 0.48; % Gravity center wrt wing apex
xcog  = (m0i*xcog0+xcogf*(FM-FM0))/m; % Gravity center wrt wing apex

%% ROTATION MATRIX

girophi   = [1,0,0;0,cos(phi),sin(phi);0,(-1).*sin(phi),cos(phi)];
girotheta = [cos(theta),0,(-1).*sin(theta);0,1,0;sin(theta),0,cos(theta)];
giropsi   = [cos(psi),sin(psi),0;(-1).*sin(psi),cos(psi),0;0,0,1];
MBH       = girophi*girotheta*giropsi; % Local horizon axes to body axes
MBHdot    = [(-1).*psidotref.*cos(theta).*sin(psi)+(-1).*thetadotref.*cos(psi).*sin(...
            theta),psidotref.*cos(psi).*cos(theta)+(-1).*thetadotref.*sin(psi).*sin(...
            theta),(-1).*thetadotref.*cos(theta);(-1).*psidotref.*cos(phi).*cos(...
            psi)+thetadotref.*cos(psi).*cos(theta).*sin(phi)+phidotref.*sin(phi).*sin(...
            psi)+phidotref.*cos(phi).*cos(psi).*sin(theta)+(-1).*psidotref.*sin(phi)...
            .*sin(psi).*sin(theta),(-1).*phidotref.*cos(psi).*sin(phi)+(-1).*...
            psidotref.*cos(phi).*sin(psi)+thetadotref.*cos(theta).*sin(phi).*sin(...
            psi)+psidotref.*cos(psi).*sin(phi).*sin(theta)+phidotref.*cos(phi).*sin(...
            psi).*sin(theta),phidotref.*cos(phi).*cos(theta)+(-1).*thetadotref.*sin(...
            phi).*sin(theta);thetadotref.*cos(phi).*cos(psi).*cos(theta)+psidotref.*...
            cos(psi).*sin(phi)+phidotref.*cos(phi).*sin(psi)+(-1).*phidotref.*cos(...
            psi).*sin(phi).*sin(theta)+(-1).*psidotref.*cos(phi).*sin(psi).*sin(...
            theta),(-1).*phidotref.*cos(phi).*cos(psi)+thetadotref.*cos(phi).*cos(...
            theta).*sin(psi)+psidotref.*sin(phi).*sin(psi)+psidotref.*cos(phi).*cos(...
            psi).*sin(theta)+(-1).*phidotref.*sin(phi).*sin(psi).*sin(theta),(-1)...
            .*phidotref.*cos(theta).*sin(phi)+(-1).*thetadotref.*cos(phi).*sin(theta)];

%% WIND PARAMETERS

uvwwind  = MBH*[Vxwind;Vywind;Vzwind];
uwind    = uvwwind(1,1);
vwind    = uvwwind(2,1);
wwind    = uvwwind(3,1);
% Wind vector derivatives are considered negligible
uvwwinddot = MBHdot*[Vxwind;Vywind;Vzwind];
uwinddot   = uvwwinddot(1,1);
vwinddot   = uvwwinddot(2,1);
wwinddot   = uvwwinddot(3,1);

%% AERODYNAMIC PARAMETERS

% Expressions of alpha, beta and V
urel     = u-uwind;
vrel     = v-vwind;
wrel     = w-wwind;
ureldot  = udotref-uwinddot;
vreldot  = vdotref-vwinddot;
wreldot  = wdotref-wwinddot;

V_total  = sqrt(urel^2+vrel^2+wrel^2);
alpha    = atan(wrel/urel);
beta     = asin(vrel/V_total);
V_dot    = (urel*ureldot+vrel*vreldot+wrel*wreldot)/V_total;
alphadot = (urel*wreldot-wrel*ureldot)/(urel^2+wrel^2);
betadot  = (vreldot*V_total-vrel*V_dot)/(V_total^2*sqrt(1-(vrel/V_total)^2));

M        = V_total/a;

% dedalpha & CD parameters
downstream = (-0.347306E1)*(0.2E1+(0.356888E2+(-0.226273E2)*M^2)^(1/2))^(-1);
oswald_f   = 0.780948; % Oswald factor
K_f        = 1/(pi*ARw*oswald_f); % Factor K of induced drag
CD0        = 0.0128115; % Parasitic drag coefficient

% Lift coefficient
CLdeltaE   = 0.222121E2.*(0.2E1+(0.339474E2+(-0.216673E2).*M.^2).^(1/2)).^(-1);
CLalphaw   = 0.298879E2.*(2+(4+0.226273E2.*(0.10001E1+(-1).*M.^2)).^(1/2)).^(-1);
CLalphat   = 0.29247E2.*(2+(4+0.216673E2.*(0.100009E1+(-1).*M.^2)).^(1/2)).^(-1);
CLalpha    = CLalphaw+CLalphat*(1+downstream)*St/Sw;
CLq        = 2*CLalphat*(St/Sw)*(xACt-xcog)/cw;
CLalphadot = -2*CLalphat*(St/Sw)*(xACt-xcog)*downstream/cw;
CL         = CLalpha*alpha+CLdeltaE*(St/Sw)*deltaE+CLq*(cw/(2*V_total))*q+...
             CLalphadot*(cw/(2*V_total))*alphadot;
% Drag coefficient
Mdiv   = 0.85;
if M < Mdiv
    CD     = CD0+K_f*CL^2;
else
    CDwave = 29.2*(M-Mdiv)^3;
    CD     = CD0+K_f*CL^2+CDwave;
end 

% Moment coefficient
CMdeltaE   = CLdeltaE*(St/Sw)*(xcog-xACt)/cw;
CMalphaw   = CLalphaw*(xcog-xACw)/cw;
CMalphat   = CLalphat*(1+downstream)*(xcog-xACt)*(St/Sw)/cw;
CMalpha    = CMalphaw+CMalphat;
CMq        = -CLq*(xACt-xcog)/cw;
CMalphadot = -CLalphadot*(xACt-xACw)/cw;
CM         = CMalpha*alpha+CMdeltaE*deltaE+CMq*(cw/(2*V_total))*q+...
             CMalphadot*(cw/(2*V_total))*alphadot;
% Lateral force coefficient
CYbeta    = -0.434283;
CYdeltaA  = 0;
CYdeltaR  = 0.0512434;
CYbetadot = 0;
CYp       = (-0.694841E-1).*(0.175E1.*cos(alpha)+(-0.54E1).*sin(alpha));
CYr       = 0.694841E-1.*(0.54E1.*cos(alpha)+0.175E1.*sin(alpha));
CY        = CYbeta*beta+CYdeltaA*deltaA+CYdeltaR*deltaR+CYbetadot*(bw/(2*V_total))*betadot...
            +CYp*(bw/(2*V_total))*p+CYr*(bw/(2*V_total))*r;
% Roll moment coefficient
CLbeta    = 0.573E2.*((-0.12E-2)+(-0.2925E-2).*(0.12E1+(0.285714E0+( ...
            0.297619E0+((-0.345238E0)+(0.327381E0+(0.102183E2+(0.426587E2+ ...
            0.257937E3.*((-0.3E0)+0.845012E0.*M)).*((-0.7E0)+0.845012E0.*M)).* ...
            ((-0.2E0)+0.845012E0.*M)).*((-0.6E0)+0.845012E0.*M)).*((-0.4E0)+ ...
            0.845012E0.*M)).*((-0.1E0)+0.845012E0.*M)).*((-0.8E0)+0.845012E0.* ...
            M))).*(0.270193E1.*deltaE.*(0.2E1+(0.339474E2+(-0.216673E2).*M.^2) ...
            .^(1/2)).^(-1)+alpha.*(0.298879E2.*(0.2E1+(0.356888E2+( ...
            -0.226273E2).*M.^2).^(1/2)).^(-1)+(2+(0.339474E2+(-0.216673E2).* ...
            M.^2).^(1/2)).^(-1).*(0.355769E1+(-0.123561E2).*(0.2E1+( ...
            0.356888E2+(-0.226273E2).*M.^2).^(1/2)).^(-1))))+0.573E2.*( ...
            0.558941E-3+(1/60).*((-0.153459E-1)+(-0.916732E-2).*(0.1275E1+( ...
            0.392857E0+(0.357143E0+(0.303571E1+((-0.14881E0)+((-0.43186E2)+(( ...
            -0.160122E3)+(0.185708E4+(0.327502E4+0.184705E5.*((-0.1226E0)+ ...
            0.845012E0.*M)).*((-0.7E0)+0.845012E0.*M)).*((-0.3E0)+0.845012E0.* ...
            M)).*((-0.75E0)+0.845012E0.*M)).*((-0.2E0)+0.845012E0.*M)).*(( ...
            -0.6E0)+0.845012E0.*M)).*((-0.4E0)+0.845012E0.*M)).*((-0.1E0)+ ...
            0.845012E0.*M)).*((-0.8E0)+0.845012E0.*M))).*pi)+(-0.347421E-1).*( ...
            0.175E1.*cos(alpha)+(-0.54E1).*sin(alpha));
CLdeltaA  = 0.169744;
CLdeltaR  = 0.453158E-2.*(0.1658E1.*cos(alpha)+(-0.605E1).*sin(alpha));
CLbetadot = 0;
CLp       = (-0.18818E-1)+(-0.355561E0).*(1+(-1).*M.^2).^(1/2);
CLr       = 0.465558E-2+0.35E0.*(1+0.612863E-1.*(0.16383E1+0.475681E1.*(1+( ...
            -0.67101E0).*M.^2).^(1/2)).*(0.327661E1+0.475681E1.*(1+( ...
            -0.67101E0).*M.^2).^(1/2)).^(-1)).^(-1).*(1+0.159594E1.*M.^2.*(1+( ...
            -0.67101E0).*M.^2).^(-1/2).*(0.16383E1+0.475681E1.*(1+(-0.67101E0) ...
            .*M.^2).^(1/2)).^(-1)+0.612863E-1.*(0.16383E1+0.475681E1.*(1+( ...
            -0.67101E0).*M.^2).^(1/2)).*(0.327661E1+0.475681E1.*(1+( ...
            -0.67101E0).*M.^2).^(1/2)).^(-1)).*(0.270193E1.*deltaE.*(0.2E1+( ...
            0.339474E2+(-0.216673E2).*M.^2).^(1/2)).^(-1)+alpha.*(0.298879E2.* ...
            (0.2E1+(0.356888E2+(-0.226273E2).*M.^2).^(1/2)).^(-1)+(2+( ...
            0.339474E2+(-0.216673E2).*M.^2).^(1/2)).^(-1).*(0.355769E1+( ...
            -0.123561E2).*(0.2E1+(0.356888E2+(-0.226273E2).*M.^2).^(1/2)).^( ...
            -1))))+0.614464E-2.*(0.175E1.*cos(alpha)+(-0.54E1).*sin(alpha)).*( ...
            0.54E1.*cos(alpha)+0.175E1.*sin(alpha));
Cl        = CLbeta*beta+CLdeltaA*deltaA+CLdeltaR*deltaR+CLbetadot*(bw/(2*V_total))*betadot...
            +CLp*(bw/(2*V_total))*p+CLr*(bw/(2*V_total))*r;
% Yaw moment coefficient
CNbeta    = (-0.21002E-1)+0.347421E-1.*(0.54E1.*cos(alpha)+0.175E1.*sin( ...
            alpha));
CNdeltaA  = 0.424361E-2.*(0.270193E1.*deltaE.*(0.2E1+(0.339474E2+(-0.216673E2) ...
            .*M.^2).^(1/2)).^(-1)+alpha.*(0.298879E2.*(0.2E1+(0.356888E2+( ...
            -0.226273E2).*M.^2).^(1/2)).^(-1)+(2+(0.339474E2+(-0.216673E2).* ...
            M.^2).^(1/2)).^(-1).*(0.355769E1+(-0.123561E2).*(0.2E1+( ...
            0.356888E2+(-0.226273E2).*M.^2).^(1/2)).^(-1))));
CNdeltaR  = (-0.453158E-2).*(0.605E1.*cos(alpha)+0.1658E1.*sin(alpha));
CNbetadot = 0;
CNp       = (-0.10627E-1).*(1+(-0.67101E0).*M.^2).^(-1/2).*(0.270193E1.* ...
            deltaE.*(0.2E1+(0.339474E2+(-0.216673E2).*M.^2).^(1/2)).^(-1)+ ...
            alpha.*(0.298879E2.*(0.2E1+(0.356888E2+(-0.226273E2).*M.^2).^(1/2) ...
            ).^(-1)+(2+(0.339474E2+(-0.216673E2).*M.^2).^(1/2)).^(-1).*( ...
            0.355769E1+(-0.123561E2).*(0.2E1+(0.356888E2+(-0.226273E2).*M.^2) ...
            .^(1/2)).^(-1))))+0.614464E-2.*((-0.175E1)+0.175E1.*cos(alpha)+( ...
            -0.54E1).*sin(alpha)).*(0.54E1.*cos(alpha)+0.175E1.*sin(alpha))+ ...
            0.353005E0.*(1+(-1).*M.^2).^(1/2).*tan(alpha)+((-0.18818E-1)+( ...
            -0.355561E0).*(1+(-1).*M.^2).^(1/2)).*tan(alpha);
CNr       = (-0.5376E-2)+(-0.5E-1).*(0.270193E1.*deltaE.*(0.2E1+(0.339474E2+ ...
            (-0.216673E2).*M.^2).^(1/2)).^(-1)+alpha.*(0.298879E2.*(0.2E1+( ...
            0.356888E2+(-0.226273E2).*M.^2).^(1/2)).^(-1)+(2+(0.339474E2+( ...
            -0.216673E2).*M.^2).^(1/2)).^(-1).*(0.355769E1+(-0.123561E2).*( ...
            0.2E1+(0.356888E2+(-0.226273E2).*M.^2).^(1/2)).^(-1)))).^2+( ...
            -0.614464E-2).*(0.54E1.*cos(alpha)+0.175E1.*sin(alpha)).^2;
CN        = CNbeta*beta+CNdeltaA*deltaA+CNdeltaR*deltaR+CNbetadot*(bw/(2*V_total))*betadot...
            +CNp*(bw/(2*V_total))*p+CNr*(bw/(2*V_total))*r;
        
%% AERODYNAMIC FORCES

Cxyz = [cos(alpha),0,(-1).*sin(alpha);0,1,0;sin(alpha),0,cos(alpha)]*...
       [-CD;CY;-CL];
Cx   = Cxyz(1,1);
Cy   = Cxyz(2,1);
Cz   = Cxyz(3,1);

FxA  = (1/2)*rho*Sw*V_total^2*Cx;
FyA  = (1/2)*rho*Sw*V_total^2*Cy;
FzA  = (1/2)*rho*Sw*V_total^2*Cz;
Lo   = (1/2)*rho*Sw*V_total^2*bw*Cl;
Mo   = (1/2)*rho*Sw*V_total^2*cw*CM;
No   = (1/2)*rho*Sw*V_total^2*bw*CN;

%% BRYAN EQUATIONS

g         = 9.81;
g_b       = MBH*[0;0;g];
V_vect    = [u;v;w]; 
Fx        = FxA+Thrust+m*g_b(1,1);
Fy        = FyA+m*g_b(2,1);
Fz        = FzA+m*g_b(3,1);
%%% Mass is considered to be constant %%%
udot      = r*v-q*w+Fx/m;
vdot      = p*w-r*u+Fy/m;
wdot      = q*u-p*v+Fz/m;

% Angular momentum (inertia moments are considered constants) %
A        = Ixx*Izz-Ixz^2;
pdot     = Lo*Izz/A+No*Ixz/A+(Ixz*(Ixx-Iyy+Izz)/A)*p*q+((Izz*(Iyy-Izz)-Ixz^2)/A)*r*q;
qdot     = Mo/Iyy+(Izz-Ixx)*p*r/Iyy+Ixz*(r^2-p^2)/Iyy;
rdot     = No*Ixx/A+Lo*Ixz/A+((Ixx*(Ixx-Iyy)+Ixz^2)/A)*p*q+(Ixz*(Iyy-Ixx-Izz)/A)*r*q;

psidot   = (r+q*tan(phi))/(cos(theta)*(cos(phi)+tan(phi)*sin(phi)));
thetadot = (q-psidot*cos(theta)*sin(phi))/cos(phi);
phidot   = p+psidot*sin(theta);

dxyz     = transpose(MBH)*V_vect;
xdot     = dxyz(1,1);
ydot     = dxyz(2,1);
zdot     = -dxyz(3,1);

Vdot     = (1/2).*(u.^2+v.^2+w.^2).^(-1/2).*(2.*u.*udot+2.*v.*vdot+2.*w.*wdot);

end
